simulink model "larix2_tuner_closedLoop"  (R2020b)
settings: Solver=FixedStepDiscrete  StartTime=0.0  StopTime=20  FixedStep=0.002  RelTol=1e-3
PostLoadFcn:
  | load('ThrustTable.mat');
  | init();
values from neighbouring files (symbols this model uses):
  blimp = inertias()    [init.m]
  eul_0 = [-45*pi/180 0 0]    [init.m]
  FLRS3_0 = [0 0 0 0]    [init.m]
  g = 9.810    (= 9.81)    [init.m]
  omega_0 = [0 0 0]    [init.m]
  pos_0 = [0 0 0]    [init.m]
  vel_0 = [0 0 0]    [init.m]
undefined symbols (not defined in the file or in its folder): DiscIntNeverNeededParam
libraries: slpidlib x10, simulink x10, sharedtransform x3, vrlib x3
(part 1 of 2)
settings Model: Creator=ac114611  LastModifiedBy=wendelin
settings DataIOCC: ExternalInput=getinputstruct(op_hover)  InitialState=getstatestruct(op_hover)  ReturnWorkspaceOutputs=off
settings OptimizationCC: DefaultParameterBehavior=Inlined  EnhancedBackFolding=on  PassReuseOutputArgsAs=Individual arguments  MaxStackSize=64  OptimizeBlockOrder=speed  DifferentSizesBufferReuse=on  EfficientTunableParamExpr=on
settings DebuggingCC: ParameterPrecisionLossMsg=none  ParameterTunabilityLossMsg=error  ArithmeticOperatorsInVariantConditions=warning
settings HardwareCC: ProdBitPerPointer=32  ProdBitPerSizeT=32  ProdBitPerPtrDiffT=32  ProdLargestAtomicInteger=Long  ProdLargestAtomicFloat=Double  ProdWordSize=32  ProdHWDeviceType=ARM Compatible->ARM Cortex  TargetBitPerLong=64  TargetBitPerPointer=64  TargetBitPerSizeT=64  TargetBitPerPtrDiffT=64  TargetLongLongMode=on  TargetIntDivRoundTo=Zero  TargetEndianess=LittleEndian  TargetWordSize=64  TargetHWDeviceType=MATLAB Host  ProdEqTarget=off
settings SFSimCC: SimUseLocalCustomCode=off  MATLABDynamicMemAlloc=off  CustomCodeUndefinedFunction=UseInterfaceOnly
settings RTWCC: Description=Embedded Coder  SystemTargetFile=ert.tlc  GenCodeOnly=on  PackageName=larix2_codegen.zip  TemplateMakefile=ert_default_tmf  RTWUseLocalCustomCode=off  Toolchain=GNU gcc/g++ | gmake (64-bit Linux)  IncludeHyperlinkInReport=on  GenerateCodeMetricsReport=on
settings CodeAppCC: ForceParamTrailComments=on  IgnoreCustomStorageClasses=off  OperatorAnnotations=on  SimulinkDataObjDesc=on  SFDataObjDesc=on  InsertBlockDesc=on
settings ERTTargetCC: TargetLangStandard=C99 (ISO)  InlinedParameterPlacement=NonHierarchical  ERTCustomFileTemplate=example_file_process.tlc

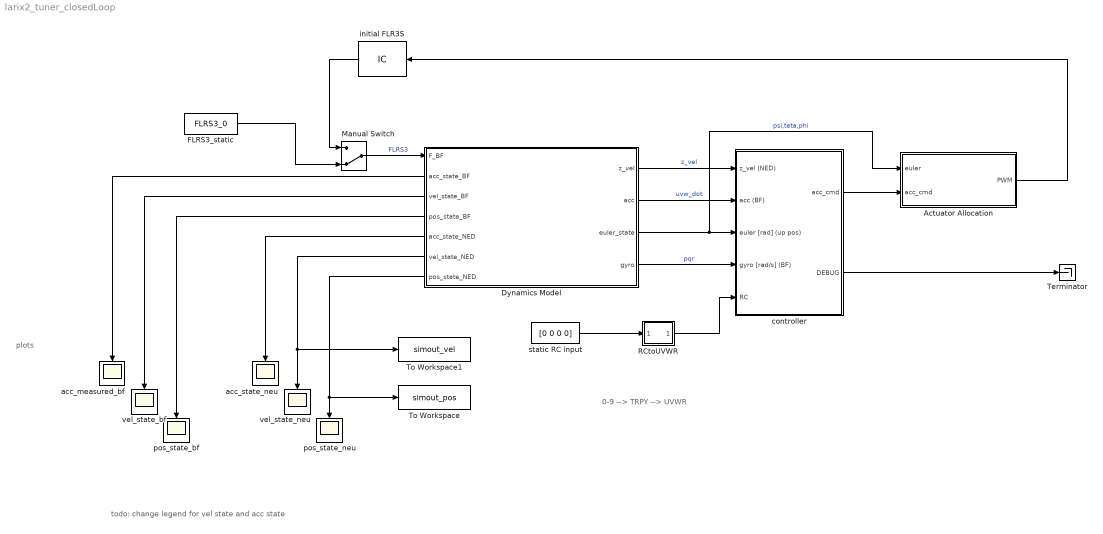
== system larix2_tuner_closedLoop ==
  note: todo: change legend for vel state and acc state
  note: plots
  note: 0-9 --> TRPY --> UVWR
  Actuator Allocation : Subsystem
  Dynamics Model : Subsystem
      settings: PortSchema="{\"entries\":[{\"content\":{\"sides\":[{\"content\":{\"connectorIds\":[\"In1\",\"Out5\",\"Out6\",\"Out7\",\"Out8\",\"Out9\",\"Out10\"]},\"type\":\"ConnectorPlacement.EquallySpacedRectSide\",\"uuid\":\"7b482eda-451f-4705-a72e-674db1e2ea8f\"},{\"content\":{\"connectorIds\":[\"Out1\",\"Out2\",\"Out3\",\"Out4\"],\"side\":\"RIGHT\"},\"type\":\"ConnectorPlacement.EquallySpacedRectSide\",\"uuid\":\"2344d3e9-2a2c-4bd3-8790-1f9d37abcd4c\"},{\"content\":{\"connectorIds\":[],\"side\":\"TOP\"},\"type\":\"ConnectorPlacement.EquallySpacedRectSide\",\"uuid\":\"13a22bb4-0a82-4477-a366-02f381e5ef07\"},{\"content\":{\"connectorIds\":[],\"side\":\"BOTTOM\"},\"type\":\"ConnectorPlacement.EquallySpacedRectSide\",\"uuid\":\"663825dc-fe4c-484f-87e0-eae3c1c76089\"},{\"content\":{\"connectorIds\":[],\"side\":\"HIDDEN\"},\"type\":\"ConnectorPlacement.EquallySpacedRectSide\",\"uuid\":\"0874c0d1-0ac2-489a-adcf-241d9ac40396\"}]},\"type\":\"ConnectorPlacement.EquallySpacedConnector\",\"uuid\":\"4f633129-49ae-43ab-aa97-bf1abe451306\"}],\"packageUris\":[\"http://schema.mathworks.com/mf0/Connector/R2020b\"],\"version\":\"1.0\"}"
  FLRS3_static : Constant  Value=FLRS3_0
  Manual Switch : ManualSwitch  CurrentSetting=0
  RCtoUVWR : Subsystem
  Terminator : Terminator
  To Workspace : ToWorkspace  VariableName=simout_pos  SaveFormat=Structure With Time  SampleTime=-1
  To Workspace1 : ToWorkspace  VariableName=simout_vel  SaveFormat=Structure With Time  SampleTime=-1
  acc_measured_bf : Scope
  acc_state_neu : Scope
  controller : Subsystem
  initial FLR3S : InitialCondition  Value=FLRS3_0
  pos_state_bf : Scope
  pos_state_neu : Scope
  static RC input : Constant  Value=[0 0 0 0]
  vel_state_bf : Scope
  vel_state_neu : Scope
  wires:
  Dynamics Model/4(gyro) -> controller/4(gyro [rad/s] (BF))  "pqr"
  Dynamics Model/2(acc) -> controller/2(acc (BF))  "uvw_dot"
  Dynamics Model/1(z_vel) -> controller/1(z_vel (NED))  "z_vel"
  Dynamics Model/3(euler_state) -> Actuator Allocation/1(euler), controller/3(euler [rad] (up pos))  "psi,teta,phi"
  Dynamics Model/6(vel_state_BF) -> vel_state_bf/1
  Dynamics Model/9(vel_state_NED) -> vel_state_neu/1, To Workspace1/1
  Dynamics Model/10(pos_state_NED) -> pos_state_neu/1, To Workspace/1
  Manual Switch/1 -> Dynamics Model/1(F_BF)  "FLRS3"
  FLRS3_static/1 -> Manual Switch/2
  initial FLR3S/1 -> Manual Switch/1
  Dynamics Model/5(acc_state_BF) -> acc_measured_bf/1
  Dynamics Model/7(pos_state_BF) -> pos_state_bf/1
  static RC input/1 -> RCtoUVWR/1(RC)
  Actuator Allocation/1(PWM) -> initial FLR3S/1
  Dynamics Model/8(acc_state_NED) -> acc_state_neu/1
  controller/2(DEBUG) -> Terminator/1
  controller/1(acc_cmd) -> Actuator Allocation/2(acc_cmd)
  RCtoUVWR/1(Out1) -> controller/5(RC)

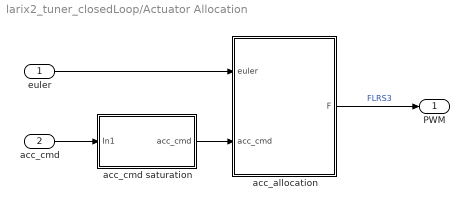
== system larix2_tuner_closedLoop/Actuator Allocation ==
  euler : Inport
  acc_cmd : Inport  Port=2
  acc_allocation : MATLAB Function  TreatAsAtomicUnit=on
  acc_cmd saturation : Subsystem
  PWM : Outport
  wires:
  acc_cmd/1 -> acc_cmd saturation/1(In1)
  acc_cmd saturation/1(acc_cmd) -> acc_allocation/2(acc_cmd)
  euler/1 -> acc_allocation/1(euler)
  acc_allocation/1(F) -> PWM/1  "FLRS3"

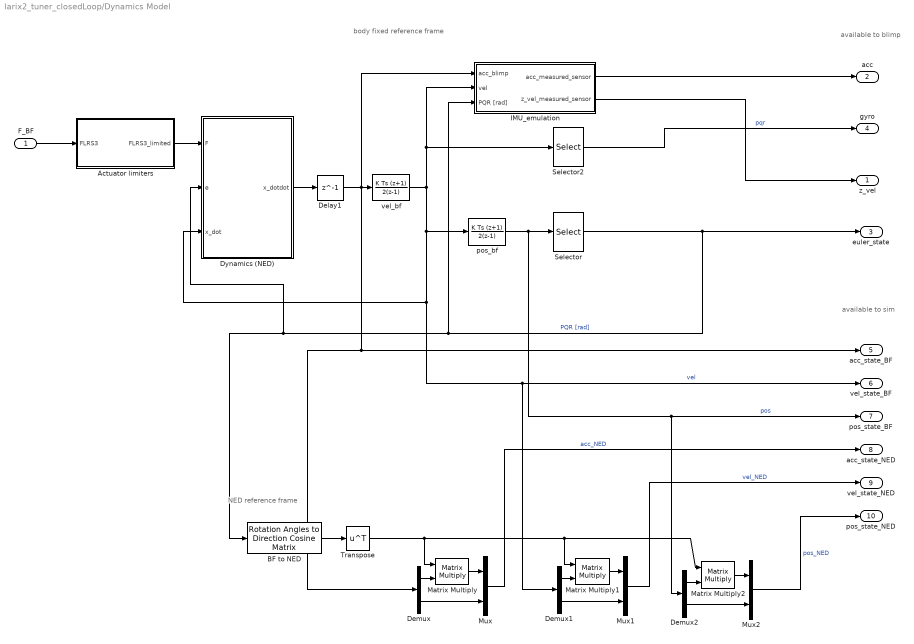
== system larix2_tuner_closedLoop/Dynamics Model ==
  note: NED reference frame
  note: body fixed reference frame
  note: available
      | to sim
  note: available
      | to blimp
  F_BF : Inport
  " BF to NED" : sharedtransform/Rotation Angles to Direction Cosine Matrix  rotationOrder=XYZ  aMode=aMode
      settings: SourceProductBaseCode=AE,PW,MT,UV,VE,VP
  Actuator limiters : Subsystem
  Delay1 : Delay  DelayLength=1  StateName=acceleration_ned
  Demux : Demux  Outputs=2
  Demux1 : Demux  Outputs=2
  Demux2 : Demux  Outputs=2
  Dynamics (NED) : MATLAB Function  TreatAsAtomicUnit=on
  IMU_emulation : Subsystem
  Matrix Multiply : Product  Multiplication=Matrix(*)
  Matrix Multiply1 : Product  Multiplication=Matrix(*)
  Matrix Multiply2 : Product  Multiplication=Matrix(*)
  Mux : Mux  Inputs=2
  Mux1 : Mux  Inputs=2
  Mux2 : Mux  Inputs=2
  Selector : Selector  InputPortWidth=6  IndexOptions=Index vector (dialog)  Indices=[4 5 6]  OutputSizes=1
  Selector2 : Selector  InputPortWidth=6  IndexOptions=Index vector (dialog)  Indices=[4 5 6]  OutputSizes=1
  Transpose : Math  Operator=transpose  SaturateOnIntegerOverflow=on
  pos_bf : DiscreteIntegrator  IntegratorMethod=Integration: Trapezoidal  InitialCondition=[pos_0,eul_0]  SampleTime=-1  StateName=position_bf  ICPrevOutput=DiscIntNeverNeededParam  ICPrevScaledInput=DiscIntNeverNeededParam
  vel_bf : DiscreteIntegrator  IntegratorMethod=Integration: Trapezoidal  InitialCondition=[vel_0,omega_0]  SampleTime=-1  StateName=velocity_bf  ICPrevOutput=DiscIntNeverNeededParam  ICPrevScaledInput=DiscIntNeverNeededParam
  z_vel : Outport  OutDataTypeStr=double
  acc : Outport  Port=2  OutDataTypeStr=double
  euler_state : Outport  Port=3  OutDataTypeStr=double
  gyro : Outport  Port=4  OutDataTypeStr=double
  acc_state_BF : Outport  Port=5
  vel_state_BF : Outport  Port=6  OutDataTypeStr=double
  pos_state_BF : Outport  Port=7
  acc_state_NED : Outport  Port=8
  vel_state_NED : Outport  Port=9
  pos_state_NED : Outport  Port=10
  wires:
  pos_bf/1 -> Demux2/1, pos_state_BF/1, Selector/1  "pos"
  vel_bf/1 -> pos_bf/1, Demux1/1, vel_state_BF/1, Dynamics (NED)/3(x_dot), Selector2/1, IMU_emulation/2(vel)  "vel"
  F_BF/1 -> Actuator limiters/1(FLRS3)
  Dynamics (NED)/1(x_dotdot) -> Delay1/1
  Selector2/1 -> gyro/1  "pqr"
  Mux2/1 -> pos_state_NED/1  "pos_NED"
  Demux/1 -> Matrix Multiply/2
  Demux/2 -> Mux/2
  Matrix Multiply/1 -> Mux/1
  Selector/1 -> Dynamics (NED)/2(e), " BF to NED"/1, IMU_emulation/3(PQR [rad]), euler_state/1  "PQR [rad]"
  Mux/1 -> acc_state_NED/1  "acc_NED"
  Mux1/1 -> vel_state_NED/1  "vel_NED"
  Delay1/1 -> Demux/1, acc_state_BF/1, vel_bf/1, IMU_emulation/1(acc_blimp)
  IMU_emulation/2(z_vel_measured_sensor) -> z_vel/1
  IMU_emulation/1(acc_measured_sensor) -> acc/1
  Demux1/1 -> Matrix Multiply1/2
  Demux1/2 -> Mux1/2
  Matrix Multiply1/1 -> Mux1/1
  Demux2/2 -> Mux2/2
  Demux2/1 -> Matrix Multiply2/2
  Matrix Multiply2/1 -> Mux2/1
  Actuator limiters/1(FLRS3_limited) -> Dynamics (NED)/1(F)
  " BF to NED"/1 -> Transpose/1
  Transpose/1 -> Matrix Multiply/1, Matrix Multiply1/1, Matrix Multiply2/1

== system larix2_tuner_closedLoop/RCtoUVWR ==
  note: uv_dot_max
      | wr_max
  note: 0-9 --> TRPY --> UVWR
  RC : Inport
  RC input safety : Subsystem
  uvwr_max : Gain  Gain=single([blimp.prp.du_input_max, blimp.prp.dv_input_max, blimp.prp.w_input_max, blimp.prp.r_input_max])
  Out1 : Outport
  wires:
  RC input safety/1(Out1) -> uvwr_max/1
  RC/1 -> RC input safety/1(RC)
  uvwr_max/1 -> Out1/1  "uvwr.desired [m/s]"

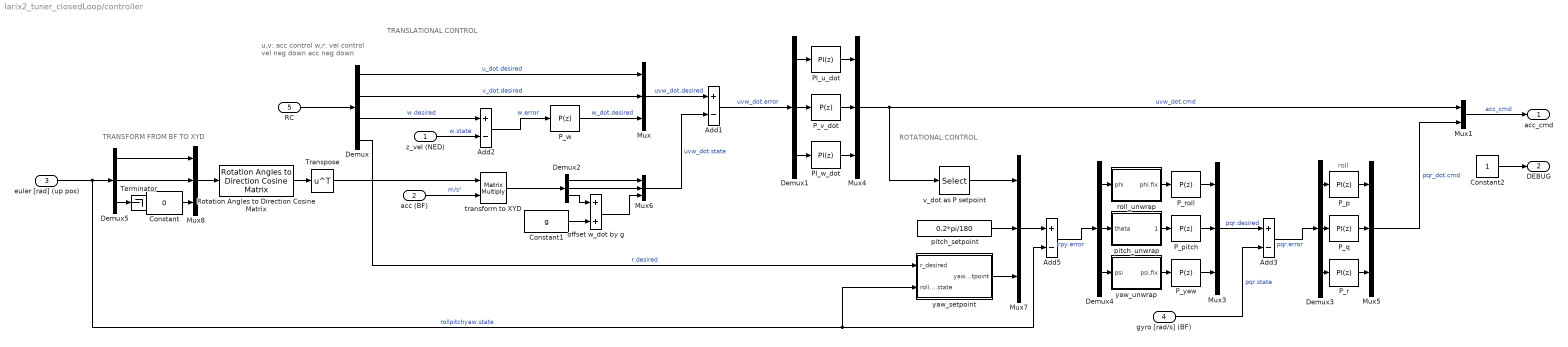
== system larix2_tuner_closedLoop/controller ==
  note: roll
  note: TRANSFORM FROM BF TO XYD
  note: u,v: acc control
      | w,r: vel control
      |
      | vel neg down
      | acc neg down
  note: TRANSLATIONAL CONTROL
  note: ROTATIONAL CONTROL
  z_vel (NED) : Inport  PortDimensions=1
  acc (BF) : Inport  Port=2  PortDimensions=3
  euler [rad] (up pos) : Inport  Port=3  PortDimensions=3
  gyro [rad/s] (BF) : Inport  Port=4  PortDimensions=3
  RC : Inport  Port=5
  Add{1..3,5} (4 alike) : Sum  Inputs=+-
  Constant : Constant  Value=0
  Constant1 : Constant  Value=g
  Constant2 : Constant
  Demux : Demux
  Demux{1..5} (5 alike) : Demux  Outputs=3
  Mux{,3..8} (7 alike) : Mux  Inputs=3
  Mux1 : Mux  Inputs=2
  PI_u_dot : slpidlib/PID Controller  Controller=PI  Form=Parallel  TimeDomain=Discrete-time  UseExternalTs=off  SampleTime=-1  IntegratorMethod=Trapezoidal  FilterMethod=Forward Euler  ControllerParametersSource=internal  P=1  I=0  D=0  UseFilter=on  N=100  TunerSelectOption=Transfer Function Based (PID Tuner App)  InitialConditionSource=internal  InitialConditionForIntegrator=0  InitialConditionForFilter=0  DifferentiatorICPrevScaledInput=0  ExternalReset=none  TrackingMode=off  Kt=1  LimitOutput=off  SatLimitsSource=internal  UpperSaturationLimit=0.4*g  LowerSaturationLimit=-0.4*g  LinearizeAsGain=off  AntiWindupMode=none  Kb=1  POutMin=[]  POutMax=[]  IOutMin=[]  IOutMax=[]  DOutMin=[]  DOutMax=[]  NOutMin=[]  NOutMax=[]  SumOutMin=[]  SumOutMax=[]  SaturationOutMin=[]  SaturationOutMax=[]  PParamMin=[]  PParamMax=[]  IParamMin=[]  IParamMax=[]  DParamMin=[]  DParamMax=[]  NParamMin=[]  NParamMax=[]  KbParamMin=[]  KbParamMax=[]  KtParamMin=[]  KtParamMax=[]  KbOutMin=[]  KbOutMax=[]  KtOutMin=[]  KtOutMax=[]  IntegratorOutMin=[]  IntegratorOutMax=[]  FilterOutMin=[]  FilterOutMax=[]  SumI1OutMin=[]  SumI1OutMax=[]  SumI2OutMin=[]  SumI2OutMax=[]  SumI3OutMin=[]  SumI3OutMax=[]  SumI4OutMin=[]  SumI4OutMax=[]  SumDOutMin=[]  SumDOutMax=[]  DifferentiatorOutMin=[]  DifferentiatorOutMax=[]  FilterDiffOutCoefMin=[]  FilterDiffOutCoefMax=[]  ReciprocalOutMin=[]  ReciprocalOutMax=[]  SumDenOutMin=[]  SumDenOutMax=[]  SumNumOutMin=[]  SumNumOutMax=[]  DivideOutMin=[]  DivideOutMax=[]  UdiffTsProdOutMin=[]  UdiffTsProdOutMax=[]  NTsProdOutMin=[]  NTsProdOutMax=[]  UintegralTsProdOutMin=[]  UintegralTsProdOutMax=[]  UngainTsProdOutMin=[]  UngainTsProdOutMax=[]  IntegratorContinuousStateAttributes=''  IntegratorStateMustResolveToSignalObject=off  IntegratorRTWStateStorageClass=Auto  FilterContinuousStateAttributes=''  FilterStateMustResolveToSignalObject=off  FilterRTWStateStorageClass=Auto  ParallelPVariant=InternalParameters  IdealPVariant=Disabled  IVariant=InternalParameters  DVariant=Disabled  IntegratorVariant=Discrete  SatVariant=Disabled  AWVariant=Passthrough  PCopyVariant=Disabled  TRVariant=Disabled  FdbkBlocksVariant=Forward  IdealPFdbkVariant=Disabled  SatFdbkVariant=Disabled  DerivativeFilterVariant=Disabled  NVariant=Disabled  NCopyVariant=Disabled_SignalSpec  FilterICVariant=Disabled  IntegratorICVariant=InternalICs  ExternalResetVariant=Disabled  TRSumVariant=Passthrough  SumFdbkVariant=Disabled  SumVariant=Sum_PI  TsampFilterVariant=InternalTs  TsampNgainVariant=Passthrough  TsampIntegralVariant=Passthrough  ExternalSaturationOutDataTypeStr=Inherit: Same as second input
  PI_w_dot : slpidlib/PID Controller  Controller=PI  Form=Parallel  TimeDomain=Discrete-time  UseExternalTs=off  SampleTime=-1  IntegratorMethod=Forward Euler  FilterMethod=Forward Euler  ControllerParametersSource=internal  P=1.8  I=1.4  D=0  UseFilter=on  N=100  TunerSelectOption=Transfer Function Based (PID Tuner App)  InitialConditionSource=internal  InitialConditionForIntegrator=1.1  InitialConditionForFilter=0  DifferentiatorICPrevScaledInput=0  ExternalReset=none  TrackingMode=off  Kt=1  LimitOutput=off  SatLimitsSource=internal  UpperSaturationLimit=inf  LowerSaturationLimit=0  LinearizeAsGain=off  AntiWindupMode=none  Kb=1  POutMin=[]  POutMax=[]  IOutMin=[]  IOutMax=[]  DOutMin=[]  DOutMax=[]  NOutMin=[]  NOutMax=[]  SumOutMin=[]  SumOutMax=[]  SaturationOutMin=[]  SaturationOutMax=[]  PParamMin=[]  PParamMax=[]  IParamMin=[]  IParamMax=[]  DParamMin=[]  DParamMax=[]  NParamMin=[]  NParamMax=[]  KbParamMin=[]  KbParamMax=[]  KtParamMin=[]  KtParamMax=[]  KbOutMin=[]  KbOutMax=[]  KtOutMin=[]  KtOutMax=[]  IntegratorOutMin=[]  IntegratorOutMax=[]  FilterOutMin=[]  FilterOutMax=[]  SumI1OutMin=[]  SumI1OutMax=[]  SumI2OutMin=[]  SumI2OutMax=[]  SumI3OutMin=[]  SumI3OutMax=[]  SumI4OutMin=[]  SumI4OutMax=[]  SumDOutMin=[]  SumDOutMax=[]  DifferentiatorOutMin=[]  DifferentiatorOutMax=[]  FilterDiffOutCoefMin=[]  FilterDiffOutCoefMax=[]  ReciprocalOutMin=[]  ReciprocalOutMax=[]  SumDenOutMin=[]  SumDenOutMax=[]  SumNumOutMin=[]  SumNumOutMax=[]  DivideOutMin=[]  DivideOutMax=[]  UdiffTsProdOutMin=[]  UdiffTsProdOutMax=[]  NTsProdOutMin=[]  NTsProdOutMax=[]  UintegralTsProdOutMin=[]  UintegralTsProdOutMax=[]  UngainTsProdOutMin=[]  UngainTsProdOutMax=[]  IntegratorContinuousStateAttributes=''  IntegratorStateMustResolveToSignalObject=off  IntegratorRTWStateStorageClass=Auto  FilterContinuousStateAttributes=''  FilterStateMustResolveToSignalObject=off  FilterRTWStateStorageClass=Auto  ParallelPVariant=InternalParameters  IdealPVariant=Disabled  IVariant=InternalParameters  DVariant=Disabled  IntegratorVariant=Discrete  SatVariant=Disabled  AWVariant=Passthrough  PCopyVariant=Disabled  TRVariant=Disabled  FdbkBlocksVariant=Forward  IdealPFdbkVariant=Disabled  SatFdbkVariant=Disabled  DerivativeFilterVariant=Disabled  NVariant=Disabled  NCopyVariant=Disabled_SignalSpec  FilterICVariant=Disabled  IntegratorICVariant=InternalICs  ExternalResetVariant=Disabled  TRSumVariant=Passthrough  SumFdbkVariant=Disabled  SumVariant=Sum_PI  TsampFilterVariant=InternalTs  TsampNgainVariant=Passthrough  TsampIntegralVariant=Passthrough  ExternalSaturationOutDataTypeStr=Inherit: Same as second input
  P_p : slpidlib/PID Controller  Controller=PI  Form=Parallel  TimeDomain=Discrete-time  UseExternalTs=off  SampleTime=-1  IntegratorMethod=Forward Euler  FilterMethod=Forward Euler  ControllerParametersSource=internal  P=1  I=0  D=0  UseFilter=on  N=100  TunerSelectOption=Transfer Function Based (PID Tuner App)  InitialConditionSource=internal  InitialConditionForIntegrator=0  InitialConditionForFilter=0  DifferentiatorICPrevScaledInput=0  ExternalReset=none  TrackingMode=off  Kt=1  LimitOutput=off  SatLimitsSource=internal  UpperSaturationLimit=inf  LowerSaturationLimit=-inf  LinearizeAsGain=on  AntiWindupMode=none  Kb=1  POutMin=[]  POutMax=[]  IOutMin=[]  IOutMax=[]  DOutMin=[]  DOutMax=[]  NOutMin=[]  NOutMax=[]  SumOutMin=[]  SumOutMax=[]  SaturationOutMin=[]  SaturationOutMax=[]  PParamMin=[]  PParamMax=[]  IParamMin=[]  IParamMax=[]  DParamMin=[]  DParamMax=[]  NParamMin=[]  NParamMax=[]  KbParamMin=[]  KbParamMax=[]  KtParamMin=[]  KtParamMax=[]  KbOutMin=[]  KbOutMax=[]  KtOutMin=[]  KtOutMax=[]  IntegratorOutMin=[]  IntegratorOutMax=[]  FilterOutMin=[]  FilterOutMax=[]  SumI1OutMin=[]  SumI1OutMax=[]  SumI2OutMin=[]  SumI2OutMax=[]  SumI3OutMin=[]  SumI3OutMax=[]  SumI4OutMin=[]  SumI4OutMax=[]  SumDOutMin=[]  SumDOutMax=[]  DifferentiatorOutMin=[]  DifferentiatorOutMax=[]  FilterDiffOutCoefMin=[]  FilterDiffOutCoefMax=[]  ReciprocalOutMin=[]  ReciprocalOutMax=[]  SumDenOutMin=[]  SumDenOutMax=[]  SumNumOutMin=[]  SumNumOutMax=[]  DivideOutMin=[]  DivideOutMax=[]  UdiffTsProdOutMin=[]  UdiffTsProdOutMax=[]  NTsProdOutMin=[]  NTsProdOutMax=[]  UintegralTsProdOutMin=[]  UintegralTsProdOutMax=[]  UngainTsProdOutMin=[]  UngainTsProdOutMax=[]  IntegratorContinuousStateAttributes=''  IntegratorStateMustResolveToSignalObject=off  IntegratorRTWStateStorageClass=Auto  FilterContinuousStateAttributes=''  FilterStateMustResolveToSignalObject=off  FilterRTWStateStorageClass=Auto  ParallelPVariant=InternalParameters  IdealPVariant=Disabled  IVariant=InternalParameters  DVariant=Disabled  IntegratorVariant=Discrete  SatVariant=Disabled  AWVariant=Passthrough  PCopyVariant=Disabled  TRVariant=Disabled  FdbkBlocksVariant=Forward  IdealPFdbkVariant=Disabled  SatFdbkVariant=Disabled  DerivativeFilterVariant=Disabled  NVariant=Disabled  NCopyVariant=Disabled_SignalSpec  FilterICVariant=Disabled  IntegratorICVariant=InternalICs  ExternalResetVariant=Disabled  TRSumVariant=Passthrough  SumFdbkVariant=Disabled  SumVariant=Sum_PI  TsampFilterVariant=InternalTs  TsampNgainVariant=Passthrough  TsampIntegralVariant=Passthrough  ExternalSaturationOutDataTypeStr=Inherit: Same as second input
  P_pitch : slpidlib/PID Controller  Controller=P  Form=Parallel  TimeDomain=Discrete-time  UseExternalTs=off  SampleTime=-1  IntegratorMethod=Forward Euler  FilterMethod=Forward Euler  ControllerParametersSource=internal  P=1  I=0  D=0  UseFilter=on  N=100  TunerSelectOption=Transfer Function Based (PID Tuner App)  InitialConditionSource=internal  InitialConditionForIntegrator=0  InitialConditionForFilter=0  DifferentiatorICPrevScaledInput=0  ExternalReset=none  TrackingMode=off  Kt=1  LimitOutput=off  SatLimitsSource=internal  UpperSaturationLimit=inf  LowerSaturationLimit=-inf  LinearizeAsGain=on  AntiWindupMode=none  Kb=1  POutMin=[]  POutMax=[]  IOutMin=[]  IOutMax=[]  DOutMin=[]  DOutMax=[]  NOutMin=[]  NOutMax=[]  SumOutMin=[]  SumOutMax=[]  SaturationOutMin=[]  SaturationOutMax=[]  PParamMin=[]  PParamMax=[]  IParamMin=[]  IParamMax=[]  DParamMin=[]  DParamMax=[]  NParamMin=[]  NParamMax=[]  KbParamMin=[]  KbParamMax=[]  KtParamMin=[]  KtParamMax=[]  KbOutMin=[]  KbOutMax=[]  KtOutMin=[]  KtOutMax=[]  IntegratorOutMin=[]  IntegratorOutMax=[]  FilterOutMin=[]  FilterOutMax=[]  SumI1OutMin=[]  SumI1OutMax=[]  SumI2OutMin=[]  SumI2OutMax=[]  SumI3OutMin=[]  SumI3OutMax=[]  SumI4OutMin=[]  SumI4OutMax=[]  SumDOutMin=[]  SumDOutMax=[]  DifferentiatorOutMin=[]  DifferentiatorOutMax=[]  FilterDiffOutCoefMin=[]  FilterDiffOutCoefMax=[]  ReciprocalOutMin=[]  ReciprocalOutMax=[]  SumDenOutMin=[]  SumDenOutMax=[]  SumNumOutMin=[]  SumNumOutMax=[]  DivideOutMin=[]  DivideOutMax=[]  UdiffTsProdOutMin=[]  UdiffTsProdOutMax=[]  NTsProdOutMin=[]  NTsProdOutMax=[]  UintegralTsProdOutMin=[]  UintegralTsProdOutMax=[]  UngainTsProdOutMin=[]  UngainTsProdOutMax=[]  IntegratorContinuousStateAttributes=''  IntegratorStateMustResolveToSignalObject=off  IntegratorRTWStateStorageClass=Auto  FilterContinuousStateAttributes=''  FilterStateMustResolveToSignalObject=off  FilterRTWStateStorageClass=Auto  ParallelPVariant=InternalParameters  IdealPVariant=Disabled  IVariant=Disabled  DVariant=Disabled  IntegratorVariant=Disabled  SatVariant=Disabled  AWVariant=Disabled  PCopyVariant=Disabled  TRVariant=Disabled  FdbkBlocksVariant=Forward  IdealPFdbkVariant=Disabled  SatFdbkVariant=Disabled  DerivativeFilterVariant=Disabled  NVariant=Disabled  NCopyVariant=Disabled_SignalSpec  FilterICVariant=Disabled  IntegratorICVariant=Disabled  ExternalResetVariant=Disabled  TRSumVariant=Passthrough  SumFdbkVariant=Disabled  SumVariant=Passthrough_P  TsampFilterVariant=InternalTs  TsampNgainVariant=Passthrough  TsampIntegralVariant=Disabled_SignalSpec  ExternalSaturationOutDataTypeStr=Inherit: Same as second input
  P_q : slpidlib/PID Controller  Controller=PI  Form=Parallel  TimeDomain=Discrete-time  UseExternalTs=off  SampleTime=-1  IntegratorMethod=Forward Euler  FilterMethod=Forward Euler  ControllerParametersSource=internal  P=1  I=0  D=0  UseFilter=on  N=100  TunerSelectOption=Transfer Function Based (PID Tuner App)  InitialConditionSource=internal  InitialConditionForIntegrator=0  InitialConditionForFilter=0  DifferentiatorICPrevScaledInput=0  ExternalReset=none  TrackingMode=off  Kt=1  LimitOutput=off  SatLimitsSource=internal  UpperSaturationLimit=inf  LowerSaturationLimit=-inf  LinearizeAsGain=on  AntiWindupMode=none  Kb=1  POutMin=[]  POutMax=[]  IOutMin=[]  IOutMax=[]  DOutMin=[]  DOutMax=[]  NOutMin=[]  NOutMax=[]  SumOutMin=[]  SumOutMax=[]  SaturationOutMin=[]  SaturationOutMax=[]  PParamMin=[]  PParamMax=[]  IParamMin=[]  IParamMax=[]  DParamMin=[]  DParamMax=[]  NParamMin=[]  NParamMax=[]  KbParamMin=[]  KbParamMax=[]  KtParamMin=[]  KtParamMax=[]  KbOutMin=[]  KbOutMax=[]  KtOutMin=[]  KtOutMax=[]  IntegratorOutMin=[]  IntegratorOutMax=[]  FilterOutMin=[]  FilterOutMax=[]  SumI1OutMin=[]  SumI1OutMax=[]  SumI2OutMin=[]  SumI2OutMax=[]  SumI3OutMin=[]  SumI3OutMax=[]  SumI4OutMin=[]  SumI4OutMax=[]  SumDOutMin=[]  SumDOutMax=[]  DifferentiatorOutMin=[]  DifferentiatorOutMax=[]  FilterDiffOutCoefMin=[]  FilterDiffOutCoefMax=[]  ReciprocalOutMin=[]  ReciprocalOutMax=[]  SumDenOutMin=[]  SumDenOutMax=[]  SumNumOutMin=[]  SumNumOutMax=[]  DivideOutMin=[]  DivideOutMax=[]  UdiffTsProdOutMin=[]  UdiffTsProdOutMax=[]  NTsProdOutMin=[]  NTsProdOutMax=[]  UintegralTsProdOutMin=[]  UintegralTsProdOutMax=[]  UngainTsProdOutMin=[]  UngainTsProdOutMax=[]  IntegratorContinuousStateAttributes=''  IntegratorStateMustResolveToSignalObject=off  IntegratorRTWStateStorageClass=Auto  FilterContinuousStateAttributes=''  FilterStateMustResolveToSignalObject=off  FilterRTWStateStorageClass=Auto  ParallelPVariant=InternalParameters  IdealPVariant=Disabled  IVariant=InternalParameters  DVariant=Disabled  IntegratorVariant=Discrete  SatVariant=Disabled  AWVariant=Passthrough  PCopyVariant=Disabled  TRVariant=Disabled  FdbkBlocksVariant=Forward  IdealPFdbkVariant=Disabled  SatFdbkVariant=Disabled  DerivativeFilterVariant=Disabled  NVariant=Disabled  NCopyVariant=Disabled_SignalSpec  FilterICVariant=Disabled  IntegratorICVariant=InternalICs  ExternalResetVariant=Disabled  TRSumVariant=Passthrough  SumFdbkVariant=Disabled  SumVariant=Sum_PI  TsampFilterVariant=InternalTs  TsampNgainVariant=Passthrough  TsampIntegralVariant=Passthrough  ExternalSaturationOutDataTypeStr=Inherit: Same as second input
  P_r : slpidlib/PID Controller  Controller=PI  Form=Parallel  TimeDomain=Discrete-time  UseExternalTs=off  SampleTime=-1  IntegratorMethod=Forward Euler  FilterMethod=Forward Euler  ControllerParametersSource=internal  P=0.7  I=0.5  D=0  UseFilter=on  N=100  TunerSelectOption=Transfer Function Based (PID Tuner App)  InitialConditionSource=internal  InitialConditionForIntegrator=0  InitialConditionForFilter=0  DifferentiatorICPrevScaledInput=0  ExternalReset=none  TrackingMode=off  Kt=1  LimitOutput=off  SatLimitsSource=internal  UpperSaturationLimit=inf  LowerSaturationLimit=-inf  LinearizeAsGain=on  AntiWindupMode=none  Kb=1  POutMin=[]  POutMax=[]  IOutMin=[]  IOutMax=[]  DOutMin=[]  DOutMax=[]  NOutMin=[]  NOutMax=[]  SumOutMin=[]  SumOutMax=[]  SaturationOutMin=[]  SaturationOutMax=[]  PParamMin=[]  PParamMax=[]  IParamMin=[]  IParamMax=[]  DParamMin=[]  DParamMax=[]  NParamMin=[]  NParamMax=[]  KbParamMin=[]  KbParamMax=[]  KtParamMin=[]  KtParamMax=[]  KbOutMin=[]  KbOutMax=[]  KtOutMin=[]  KtOutMax=[]  IntegratorOutMin=[]  IntegratorOutMax=[]  FilterOutMin=[]  FilterOutMax=[]  SumI1OutMin=[]  SumI1OutMax=[]  SumI2OutMin=[]  SumI2OutMax=[]  SumI3OutMin=[]  SumI3OutMax=[]  SumI4OutMin=[]  SumI4OutMax=[]  SumDOutMin=[]  SumDOutMax=[]  DifferentiatorOutMin=[]  DifferentiatorOutMax=[]  FilterDiffOutCoefMin=[]  FilterDiffOutCoefMax=[]  ReciprocalOutMin=[]  ReciprocalOutMax=[]  SumDenOutMin=[]  SumDenOutMax=[]  SumNumOutMin=[]  SumNumOutMax=[]  DivideOutMin=[]  DivideOutMax=[]  UdiffTsProdOutMin=[]  UdiffTsProdOutMax=[]  NTsProdOutMin=[]  NTsProdOutMax=[]  UintegralTsProdOutMin=[]  UintegralTsProdOutMax=[]  UngainTsProdOutMin=[]  UngainTsProdOutMax=[]  IntegratorContinuousStateAttributes=''  IntegratorStateMustResolveToSignalObject=off  IntegratorRTWStateStorageClass=Auto  FilterContinuousStateAttributes=''  FilterStateMustResolveToSignalObject=off  FilterRTWStateStorageClass=Auto  ParallelPVariant=InternalParameters  IdealPVariant=Disabled  IVariant=InternalParameters  DVariant=Disabled  IntegratorVariant=Discrete  SatVariant=Disabled  AWVariant=Passthrough  PCopyVariant=Disabled  TRVariant=Disabled  FdbkBlocksVariant=Forward  IdealPFdbkVariant=Disabled  SatFdbkVariant=Disabled  DerivativeFilterVariant=Disabled  NVariant=Disabled  NCopyVariant=Disabled_SignalSpec  FilterICVariant=Disabled  IntegratorICVariant=InternalICs  ExternalResetVariant=Disabled  TRSumVariant=Passthrough  SumFdbkVariant=Disabled  SumVariant=Sum_PI  TsampFilterVariant=InternalTs  TsampNgainVariant=Passthrough  TsampIntegralVariant=Passthrough  ExternalSaturationOutDataTypeStr=Inherit: Same as second input
  P_roll : slpidlib/PID Controller  Controller=P  Form=Parallel  TimeDomain=Discrete-time  UseExternalTs=off  SampleTime=-1  IntegratorMethod=Forward Euler  FilterMethod=Forward Euler  ControllerParametersSource=internal  P=0  I=0  D=0  UseFilter=on  N=100  TunerSelectOption=Transfer Function Based (PID Tuner App)  InitialConditionSource=internal  InitialConditionForIntegrator=0  InitialConditionForFilter=0  DifferentiatorICPrevScaledInput=0  ExternalReset=none  TrackingMode=off  Kt=1  LimitOutput=off  SatLimitsSource=internal  UpperSaturationLimit=inf  LowerSaturationLimit=-inf  LinearizeAsGain=on  AntiWindupMode=none  Kb=1  POutMin=[]  POutMax=[]  IOutMin=[]  IOutMax=[]  DOutMin=[]  DOutMax=[]  NOutMin=[]  NOutMax=[]  SumOutMin=[]  SumOutMax=[]  SaturationOutMin=[]  SaturationOutMax=[]  PParamMin=[]  PParamMax=[]  IParamMin=[]  IParamMax=[]  DParamMin=[]  DParamMax=[]  NParamMin=[]  NParamMax=[]  KbParamMin=[]  KbParamMax=[]  KtParamMin=[]  KtParamMax=[]  KbOutMin=[]  KbOutMax=[]  KtOutMin=[]  KtOutMax=[]  IntegratorOutMin=[]  IntegratorOutMax=[]  FilterOutMin=[]  FilterOutMax=[]  SumI1OutMin=[]  SumI1OutMax=[]  SumI2OutMin=[]  SumI2OutMax=[]  SumI3OutMin=[]  SumI3OutMax=[]  SumI4OutMin=[]  SumI4OutMax=[]  SumDOutMin=[]  SumDOutMax=[]  DifferentiatorOutMin=[]  DifferentiatorOutMax=[]  FilterDiffOutCoefMin=[]  FilterDiffOutCoefMax=[]  ReciprocalOutMin=[]  ReciprocalOutMax=[]  SumDenOutMin=[]  SumDenOutMax=[]  SumNumOutMin=[]  SumNumOutMax=[]  DivideOutMin=[]  DivideOutMax=[]  UdiffTsProdOutMin=[]  UdiffTsProdOutMax=[]  NTsProdOutMin=[]  NTsProdOutMax=[]  UintegralTsProdOutMin=[]  UintegralTsProdOutMax=[]  UngainTsProdOutMin=[]  UngainTsProdOutMax=[]  IntegratorContinuousStateAttributes=''  IntegratorStateMustResolveToSignalObject=off  IntegratorRTWStateStorageClass=Auto  FilterContinuousStateAttributes=''  FilterStateMustResolveToSignalObject=off  FilterRTWStateStorageClass=Auto  ParallelPVariant=InternalParameters  IdealPVariant=Disabled  IVariant=Disabled  DVariant=Disabled  IntegratorVariant=Disabled  SatVariant=Disabled  AWVariant=Disabled  PCopyVariant=Disabled  TRVariant=Disabled  FdbkBlocksVariant=Forward  IdealPFdbkVariant=Disabled  SatFdbkVariant=Disabled  DerivativeFilterVariant=Disabled  NVariant=Disabled  NCopyVariant=Disabled_SignalSpec  FilterICVariant=Disabled  IntegratorICVariant=Disabled  ExternalResetVariant=Disabled  TRSumVariant=Passthrough  SumFdbkVariant=Disabled  SumVariant=Passthrough_P  TsampFilterVariant=InternalTs  TsampNgainVariant=Passthrough  TsampIntegralVariant=Disabled_SignalSpec  ExternalSaturationOutDataTypeStr=Inherit: Same as second input
  P_v_dot : slpidlib/PID Controller  Controller=P  Form=Parallel  TimeDomain=Discrete-time  UseExternalTs=off  SampleTime=-1  IntegratorMethod=Forward Euler  FilterMethod=Forward Euler  ControllerParametersSource=internal  P=2.5 *pi/180  I=1  D=0  UseFilter=on  N=100  TunerSelectOption=Transfer Function Based (PID Tuner App)  InitialConditionSource=internal  InitialConditionForIntegrator=0  InitialConditionForFilter=0  DifferentiatorICPrevScaledInput=0  ExternalReset=none  TrackingMode=off  Kt=1  LimitOutput=off  SatLimitsSource=internal  UpperSaturationLimit=inf  LowerSaturationLimit=-inf  LinearizeAsGain=on  AntiWindupMode=none  Kb=1  POutMin=[]  POutMax=[]  IOutMin=[]  IOutMax=[]  DOutMin=[]  DOutMax=[]  NOutMin=[]  NOutMax=[]  SumOutMin=[]  SumOutMax=[]  SaturationOutMin=[]  SaturationOutMax=[]  PParamMin=[]  PParamMax=[]  IParamMin=[]  IParamMax=[]  DParamMin=[]  DParamMax=[]  NParamMin=[]  NParamMax=[]  KbParamMin=[]  KbParamMax=[]  KtParamMin=[]  KtParamMax=[]  KbOutMin=[]  KbOutMax=[]  KtOutMin=[]  KtOutMax=[]  IntegratorOutMin=[]  IntegratorOutMax=[]  FilterOutMin=[]  FilterOutMax=[]  SumI1OutMin=[]  SumI1OutMax=[]  SumI2OutMin=[]  SumI2OutMax=[]  SumI3OutMin=[]  SumI3OutMax=[]  SumI4OutMin=[]  SumI4OutMax=[]  SumDOutMin=[]  SumDOutMax=[]  DifferentiatorOutMin=[]  DifferentiatorOutMax=[]  FilterDiffOutCoefMin=[]  FilterDiffOutCoefMax=[]  ReciprocalOutMin=[]  ReciprocalOutMax=[]  SumDenOutMin=[]  SumDenOutMax=[]  SumNumOutMin=[]  SumNumOutMax=[]  DivideOutMin=[]  DivideOutMax=[]  UdiffTsProdOutMin=[]  UdiffTsProdOutMax=[]  NTsProdOutMin=[]  NTsProdOutMax=[]  UintegralTsProdOutMin=[]  UintegralTsProdOutMax=[]  UngainTsProdOutMin=[]  UngainTsProdOutMax=[]  IntegratorContinuousStateAttributes=''  IntegratorStateMustResolveToSignalObject=off  IntegratorRTWStateStorageClass=Auto  FilterContinuousStateAttributes=''  FilterStateMustResolveToSignalObject=off  FilterRTWStateStorageClass=Auto  ParallelPVariant=InternalParameters  IdealPVariant=Disabled  IVariant=Disabled  DVariant=Disabled  IntegratorVariant=Disabled  SatVariant=Disabled  AWVariant=Disabled  PCopyVariant=Disabled  TRVariant=Disabled  FdbkBlocksVariant=Forward  IdealPFdbkVariant=Disabled  SatFdbkVariant=Disabled  DerivativeFilterVariant=Disabled  NVariant=Disabled  NCopyVariant=Disabled_SignalSpec  FilterICVariant=Disabled  IntegratorICVariant=Disabled  ExternalResetVariant=Disabled  TRSumVariant=Passthrough  SumFdbkVariant=Disabled  SumVariant=Passthrough_P  TsampFilterVariant=InternalTs  TsampNgainVariant=Passthrough  TsampIntegralVariant=Disabled_SignalSpec  ExternalSaturationOutDataTypeStr=Inherit: Same as second input
  P_w : slpidlib/PID Controller  Controller=P  Form=Parallel  TimeDomain=Discrete-time  UseExternalTs=off  SampleTime=-1  IntegratorMethod=Forward Euler  FilterMethod=Forward Euler  ControllerParametersSource=internal  P=1.3  I=0  D=0  UseFilter=on  N=100  TunerSelectOption=Transfer Function Based (PID Tuner App)  InitialConditionSource=internal  InitialConditionForIntegrator=0  InitialConditionForFilter=0  DifferentiatorICPrevScaledInput=0  ExternalReset=none  TrackingMode=off  Kt=1  LimitOutput=off  SatLimitsSource=internal  UpperSaturationLimit=inf  LowerSaturationLimit=-inf  LinearizeAsGain=off  AntiWindupMode=none  Kb=1  POutMin=[]  POutMax=[]  IOutMin=[]  IOutMax=[]  DOutMin=[]  DOutMax=[]  NOutMin=[]  NOutMax=[]  SumOutMin=[]  SumOutMax=[]  SaturationOutMin=[]  SaturationOutMax=[]  PParamMin=[]  PParamMax=[]  IParamMin=[]  IParamMax=[]  DParamMin=[]  DParamMax=[]  NParamMin=[]  NParamMax=[]  KbParamMin=[]  KbParamMax=[]  KtParamMin=[]  KtParamMax=[]  KbOutMin=[]  KbOutMax=[]  KtOutMin=[]  KtOutMax=[]  IntegratorOutMin=[]  IntegratorOutMax=[]  FilterOutMin=[]  FilterOutMax=[]  SumI1OutMin=[]  SumI1OutMax=[]  SumI2OutMin=[]  SumI2OutMax=[]  SumI3OutMin=[]  SumI3OutMax=[]  SumI4OutMin=[]  SumI4OutMax=[]  SumDOutMin=[]  SumDOutMax=[]  DifferentiatorOutMin=[]  DifferentiatorOutMax=[]  FilterDiffOutCoefMin=[]  FilterDiffOutCoefMax=[]  ReciprocalOutMin=[]  ReciprocalOutMax=[]  SumDenOutMin=[]  SumDenOutMax=[]  SumNumOutMin=[]  SumNumOutMax=[]  DivideOutMin=[]  DivideOutMax=[]  UdiffTsProdOutMin=[]  UdiffTsProdOutMax=[]  NTsProdOutMin=[]  NTsProdOutMax=[]  UintegralTsProdOutMin=[]  UintegralTsProdOutMax=[]  UngainTsProdOutMin=[]  UngainTsProdOutMax=[]  IntegratorContinuousStateAttributes=''  IntegratorStateMustResolveToSignalObject=off  IntegratorRTWStateStorageClass=Auto  FilterContinuousStateAttributes=''  FilterStateMustResolveToSignalObject=off  FilterRTWStateStorageClass=Auto  ParallelPVariant=InternalParameters  IdealPVariant=Disabled  IVariant=Disabled  DVariant=Disabled  IntegratorVariant=Disabled  SatVariant=Disabled  AWVariant=Disabled  PCopyVariant=Disabled  TRVariant=Disabled  FdbkBlocksVariant=Forward  IdealPFdbkVariant=Disabled  SatFdbkVariant=Disabled  DerivativeFilterVariant=Disabled  NVariant=Disabled  NCopyVariant=Disabled_SignalSpec  FilterICVariant=Disabled  IntegratorICVariant=Disabled  ExternalResetVariant=Disabled  TRSumVariant=Passthrough  SumFdbkVariant=Disabled  SumVariant=Passthrough_P  TsampFilterVariant=InternalTs  TsampNgainVariant=Passthrough  TsampIntegralVariant=Disabled_SignalSpec  ExternalSaturationOutDataTypeStr=Inherit: Same as second input
  P_yaw : slpidlib/PID Controller  Controller=P  Form=Parallel  TimeDomain=Discrete-time  UseExternalTs=off  SampleTime=-1  IntegratorMethod=Forward Euler  FilterMethod=Forward Euler  ControllerParametersSource=internal  P=1.2  I=0  D=0  UseFilter=on  N=100  TunerSelectOption=Transfer Function Based (PID Tuner App)  InitialConditionSource=internal  InitialConditionForIntegrator=0  InitialConditionForFilter=0  DifferentiatorICPrevScaledInput=0  ExternalReset=none  TrackingMode=off  Kt=1  LimitOutput=off  SatLimitsSource=internal  UpperSaturationLimit=inf  LowerSaturationLimit=-inf  LinearizeAsGain=on  AntiWindupMode=none  Kb=1  POutMin=[]  POutMax=[]  IOutMin=[]  IOutMax=[]  DOutMin=[]  DOutMax=[]  NOutMin=[]  NOutMax=[]  SumOutMin=[]  SumOutMax=[]  SaturationOutMin=[]  SaturationOutMax=[]  PParamMin=[]  PParamMax=[]  IParamMin=[]  IParamMax=[]  DParamMin=[]  DParamMax=[]  NParamMin=[]  NParamMax=[]  KbParamMin=[]  KbParamMax=[]  KtParamMin=[]  KtParamMax=[]  KbOutMin=[]  KbOutMax=[]  KtOutMin=[]  KtOutMax=[]  IntegratorOutMin=[]  IntegratorOutMax=[]  FilterOutMin=[]  FilterOutMax=[]  SumI1OutMin=[]  SumI1OutMax=[]  SumI2OutMin=[]  SumI2OutMax=[]  SumI3OutMin=[]  SumI3OutMax=[]  SumI4OutMin=[]  SumI4OutMax=[]  SumDOutMin=[]  SumDOutMax=[]  DifferentiatorOutMin=[]  DifferentiatorOutMax=[]  FilterDiffOutCoefMin=[]  FilterDiffOutCoefMax=[]  ReciprocalOutMin=[]  ReciprocalOutMax=[]  SumDenOutMin=[]  SumDenOutMax=[]  SumNumOutMin=[]  SumNumOutMax=[]  DivideOutMin=[]  DivideOutMax=[]  UdiffTsProdOutMin=[]  UdiffTsProdOutMax=[]  NTsProdOutMin=[]  NTsProdOutMax=[]  UintegralTsProdOutMin=[]  UintegralTsProdOutMax=[]  UngainTsProdOutMin=[]  UngainTsProdOutMax=[]  IntegratorContinuousStateAttributes=''  IntegratorStateMustResolveToSignalObject=off  IntegratorRTWStateStorageClass=Auto  FilterContinuousStateAttributes=''  FilterStateMustResolveToSignalObject=off  FilterRTWStateStorageClass=Auto  ParallelPVariant=InternalParameters  IdealPVariant=Disabled  IVariant=Disabled  DVariant=Disabled  IntegratorVariant=Disabled  SatVariant=Disabled  AWVariant=Disabled  PCopyVariant=Disabled  TRVariant=Disabled  FdbkBlocksVariant=Forward  IdealPFdbkVariant=Disabled  SatFdbkVariant=Disabled  DerivativeFilterVariant=Disabled  NVariant=Disabled  NCopyVariant=Disabled_SignalSpec  FilterICVariant=Disabled  IntegratorICVariant=Disabled  ExternalResetVariant=Disabled  TRSumVariant=Passthrough  SumFdbkVariant=Disabled  SumVariant=Passthrough_P  TsampFilterVariant=InternalTs  TsampNgainVariant=Passthrough  TsampIntegralVariant=Disabled_SignalSpec  ExternalSaturationOutDataTypeStr=Inherit: Same as second input
  Rotation Angles to Direction Cosine Matrix : sharedtransform/Rotation Angles to Direction Cosine Matrix  rotationOrder=XYZ  aMode=aMode
      settings: SourceProductBaseCode=AE,PW,MT,UV,VE,VP
  Terminator : Terminator
  Transpose : Math  Operator=transpose  SaturateOnIntegerOverflow=on
  offset w_dot by g : Sum
  pitch_setpoint : Constant  Value=0.2*pi/180
  pitch_unwrap : Subsystem
  roll_unwrap : Subsystem
  transform to XYD : Product  Multiplication=Matrix(*)
  v_dot as P setpoint : Selector  InputPortWidth=3  IndexOptions=Index vector (dialog)  Indices=[2]  OutputSizes=1
  yaw_setpoint : Subsystem
  yaw_unwrap : Subsystem
  acc_cmd : Outport
  DEBUG : Outport  Port=2
  wires:
  Mux1/1 -> acc_cmd/1  "acc_cmd"
  P_r/1 -> Mux5/3
  Mux6/1 -> Add1/2  "uvw_dot.state"
  Demux/1 -> Mux/1  "u_dot.desired"
  offset w_dot by g/1 -> Mux6/3
  Add3/1 -> Demux3/1  "pqr.error"
  Demux2/3 -> offset w_dot by g/1
  Add2/1 -> P_w/1  "w.error"
  Demux3/2 -> P_q/1
  P_p/1 -> Mux5/1
  Demux/4 -> yaw_setpoint/1(r_desired)  "r.desired"
  Demux1/3 -> PI_w_dot/1
  Constant1/1 -> offset w_dot by g/2
  Demux/2 -> Mux/2  "v_dot.desired"
  P_w/1 -> Mux/3  "w_dot.desired"
  Mux4/1 -> v_dot as P setpoint/1, Mux1/1  "uvw_dot.cmd"
  Demux3/3 -> P_r/1
  z_vel (NED)/1 -> Add2/2  "w.state"
  Demux3/1 -> P_p/1
  PI_w_dot/1 -> Mux4/3
  P_q/1 -> Mux5/2
  gyro [rad/s] (BF)/1 -> Add3/2  "pqr.state"
  euler [rad] (up pos)/1 -> Add5/2, yaw_setpoint/2(rollpitchyaw.state), Demux5/1  "rollpitchyaw.state"
  PI_u_dot/1 -> Mux4/1
  Demux1/2 -> P_v_dot/1
  Mux/1 -> Add1/1  "uvw_dot.desired"
  RC/1 -> Demux/1
  Mux5/1 -> Mux1/2  "pqr_dot.cmd"
  Add5/1 -> Demux4/1  "rpy.error"
  Add1/1 -> Demux1/1  "uvw_dot.error"
  acc (BF)/1 -> transform to XYD/2  "m/s²"
  Demux/3 -> Add2/1  "w.desired"
  Demux4/2 -> pitch_unwrap/1(theta)
  P_roll/1 -> Mux3/1
  Demux1/1 -> PI_u_dot/1
  Mux3/1 -> Add3/1  "pqr.desired"
  P_pitch/1 -> Mux3/2
  pitch_setpoint/1 -> Mux7/2
  Mux7/1 -> Add5/1
  Demux5/1 -> Mux8/1
  Demux5/2 -> Mux8/2
  Demux5/3 -> Terminator/1
  Constant/1 -> Mux8/3
  Mux8/1 -> Rotation Angles to Direction Cosine Matrix/1
  transform to XYD/1 -> Demux2/1
  Demux2/2 -> Mux6/2
  yaw_setpoint/1(yaw_setpoint) -> Mux7/3
  Demux4/3 -> yaw_unwrap/1(psi)
  P_yaw/1 -> Mux3/3
  yaw_unwrap/1(psi.fix) -> P_yaw/1
  Demux4/1 -> roll_unwrap/1(phi)
  P_v_dot/1 -> Mux4/2
  Demux2/1 -> Mux6/1
  v_dot as P setpoint/1 -> Mux7/1
  Constant2/1 -> DEBUG/1
  Rotation Angles to Direction Cosine Matrix/1 -> Transpose/1
  Transpose/1 -> transform to XYD/1
  pitch_unwrap/1(theta.fix) -> P_pitch/1
  roll_unwrap/1(phi.fix) -> P_roll/1

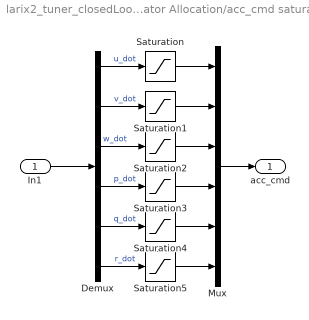
== system larix2_tuner_closedLoop/Actuator Allocation/acc_cmd saturation ==
  In1 : Inport
  Demux : Demux  Outputs=6
  Mux : Mux  Inputs=6
  Saturation : Saturate  UpperLimit=blimp.prp.du_max  LowerLimit=-blimp.prp.du_max
  Saturation1 : Saturate  UpperLimit=blimp.prp.dv_max  LowerLimit=-blimp.prp.dv_max
  Saturation2 : Saturate  UpperLimit=blimp.prp.dw_max  LowerLimit=-blimp.prp.dw_max
  Saturation3 : Saturate  UpperLimit=blimp.prp.dp_max  LowerLimit=-blimp.prp.dp_max
  Saturation4 : Saturate  UpperLimit=blimp.prp.dq_max  LowerLimit=-blimp.prp.dq_max
  Saturation5 : Saturate  UpperLimit=blimp.prp.dr_max  LowerLimit=-blimp.prp.dr_max
  acc_cmd : Outport
  wires:
  In1/1 -> Demux/1
  Mux/1 -> acc_cmd/1
  Demux/1 -> Saturation/1  "u_dot"
  Saturation/1 -> Mux/1
  Demux/2 -> Saturation1/1  "v_dot"
  Saturation1/1 -> Mux/2
  Demux/3 -> Saturation2/1  "w_dot"
  Saturation2/1 -> Mux/3
  Demux/4 -> Saturation3/1  "p_dot"
  Saturation3/1 -> Mux/4
  Demux/5 -> Saturation4/1  "q_dot"
  Saturation4/1 -> Mux/5
  Demux/6 -> Saturation5/1  "r_dot"
  Saturation5/1 -> Mux/6

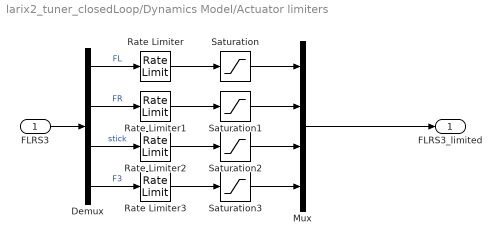
== system larix2_tuner_closedLoop/Dynamics Model/Actuator limiters ==
  FLRS3 : Inport
  Demux : Demux
  Mux : Mux
  Rate Limiter : RateLimiter  RisingSlewLimit=blimp.prp.dFLR_max  FallingSlewLimit=-blimp.prp.dFLR_max  SampleTimeMode=inherited
  Rate Limiter1 : RateLimiter  RisingSlewLimit=blimp.prp.dFLR_max  FallingSlewLimit=-blimp.prp.dFLR_max  SampleTimeMode=inherited
  Rate Limiter2 : RateLimiter  RisingSlewLimit=blimp.prp.dstick_max  FallingSlewLimit=-blimp.prp.dstick_max  SampleTimeMode=inherited
  Rate Limiter3 : RateLimiter  RisingSlewLimit=blimp.prp.dF3_max  FallingSlewLimit=-blimp.prp.dF3_max  SampleTimeMode=inherited
  Saturation : Saturate  UpperLimit=blimp.prp.FL_max  LowerLimit=blimp.prp.FL_min
  Saturation1 : Saturate  UpperLimit=blimp.prp.FR_max  LowerLimit=blimp.prp.FR_min
  Saturation2 : Saturate  UpperLimit=blimp.prp.stick_max  LowerLimit=blimp.prp.stick_min
  Saturation3 : Saturate  UpperLimit=blimp.prp.FB_max  LowerLimit=blimp.prp.FB_min
  FLRS3_limited : Outport
  wires:
  FLRS3/1 -> Demux/1
  Demux/1 -> Rate Limiter/1  "FL"
  Rate Limiter/1 -> Saturation/1
  Demux/2 -> Rate Limiter1/1  "FR"
  Rate Limiter1/1 -> Saturation1/1
  Demux/3 -> Rate Limiter2/1  "stick"
  Rate Limiter2/1 -> Saturation2/1
  Demux/4 -> Rate Limiter3/1  "F3"
  Rate Limiter3/1 -> Saturation3/1
  Mux/1 -> FLRS3_limited/1
  Saturation/1 -> Mux/1
  Saturation1/1 -> Mux/2
  Saturation2/1 -> Mux/3
  Saturation3/1 -> Mux/4

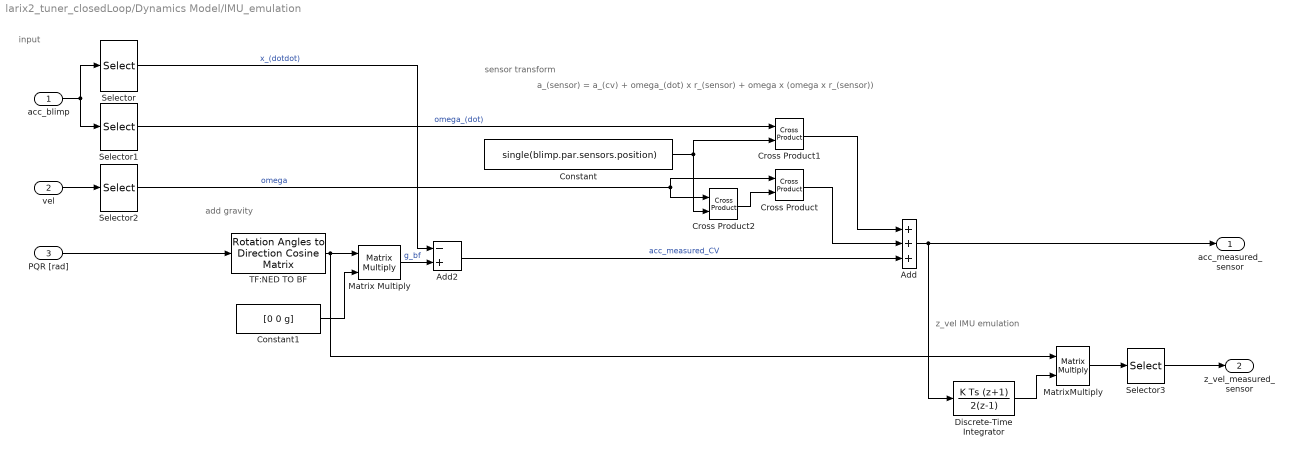
== system larix2_tuner_closedLoop/Dynamics Model/IMU_emulation ==
  note: z_vel IMU emulation
  note: a_(sensor) = a_(cv) + omega_(dot) x r_(sensor) + omega x (omega x r_(sensor))
  note: input
  note: add gravity
  note: sensor transform
  acc_blimp : Inport
  vel : Inport  Port=2
  PQR [rad] : Inport  Port=3
  Add : Sum  Inputs=+++
  Add2 : Sum  Inputs=-+
  Constant : Constant  Value=single(blimp.par.sensors.position)
  Constant1 : Constant  Value=[0 0 g]
  Cross Product : vrlib/Utilities/Cross Product
  Cross Product1 : vrlib/Utilities/Cross Product
  Cross Product2 : vrlib/Utilities/Cross Product
  Discrete-Time Integrator : DiscreteIntegrator  IntegratorMethod=Integration: Trapezoidal  gainval=1  SampleTime=-1  ICPrevOutput=DiscIntNeverNeededParam  ICPrevScaledInput=DiscIntNeverNeededParam
  Matrix Multiply : Product  Multiplication=Matrix(*)
  MatrixMultiply : Product  Multiplication=Matrix(*)
  Selector : Selector  InputPortWidth=6  IndexOptions=Index vector (dialog)  Indices=[1 2 3]  OutputSizes=1
  Selector1 : Selector  InputPortWidth=6  IndexOptions=Index vector (dialog)  Indices=[4 5 6]  OutputSizes=1
  Selector2 : Selector  InputPortWidth=6  IndexOptions=Index vector (dialog)  Indices=[4 5 6]  OutputSizes=1
  Selector3 : Selector  InputPortWidth=3  IndexOptions=Index vector (dialog)  Indices=[3]  OutputSizes=1
  TF:NED TO BF : sharedtransform/Rotation Angles to Direction Cosine Matrix  rotationOrder=XYZ  aMode=aMode
      settings: SourceProductBaseCode=AE,PW,MT,UV,VE,VP
  acc_measured_sensor : Outport
  z_vel_measured_sensor : Outport  Port=2
  wires:
  Add2/1 -> Add/3  "acc_measured_CV"
  Cross Product/1 -> Add/2
  Cross Product2/1 -> Cross Product/2
  Cross Product1/1 -> Add/1
  Selector/1 -> Add2/1  "x_(dotdot)"
  Constant/1 -> Cross Product1/2, Cross Product2/2
  acc_blimp/1 -> Selector1/1, Selector/1
  Constant1/1 -> Matrix Multiply/2
  Matrix Multiply/1 -> Add2/2  "g_bf"
  TF:NED TO BF/1 -> MatrixMultiply/1, Matrix Multiply/1
  PQR [rad]/1 -> TF:NED TO BF/1
  Selector1/1 -> Cross Product1/1  "omega_(dot)"
  vel/1 -> Selector2/1
  Selector2/1 -> Cross Product/1, Cross Product2/1  "omega"
  Add/1 -> Discrete-Time Integrator/1, acc_measured_sensor/1
  Discrete-Time Integrator/1 -> MatrixMultiply/2
  MatrixMultiply/1 -> Selector3/1
  Selector3/1 -> z_vel_measured_sensor/1

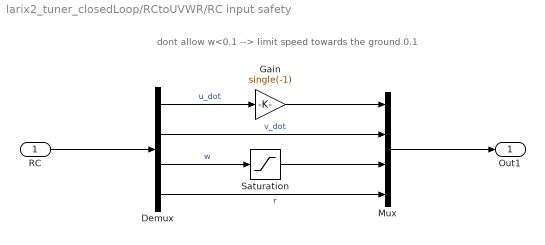
== system larix2_tuner_closedLoop/RCtoUVWR/RC input safety ==
  note: dont allow w<0.1 --> limit speed towards the ground
      |
      |  0.1
  RC : Inport
  Demux : Demux
  Gain : Gain  Gain=single(-1)
  Mux : Mux
  Saturation : Saturate  UpperLimit=1  LowerLimit=-0.2
  Out1 : Outport
  wires:
  RC/1 -> Demux/1
  Mux/1 -> Out1/1
  Demux/1 -> Gain/1  "u_dot"
  Demux/2 -> Mux/2  "v_dot"
  Demux/4 -> Mux/4  "r"
  Demux/3 -> Saturation/1  "w"
  Saturation/1 -> Mux/3
  Gain/1 -> Mux/1

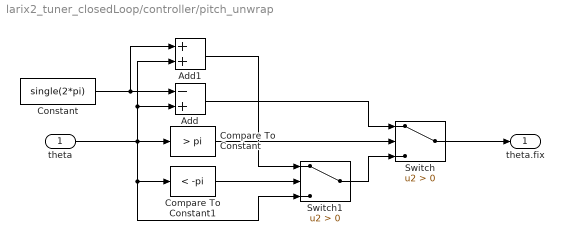
== system larix2_tuner_closedLoop/controller/pitch_unwrap ==
  theta : Inport
  Add : Sum  Inputs=-+
  Add1 : Sum
  Compare To Constant : simulink/Logic and Bit Operations/Compare To Constant  relop=>  const=pi  OutDataTypeStr=boolean
  Compare To Constant1 : simulink/Logic and Bit Operations/Compare To Constant  relop=<  const=-pi  OutDataTypeStr=boolean
  Constant : Constant  Value=single(2*pi)
  Switch : Switch  Criteria=u2 > Threshold
  Switch1 : Switch  Criteria=u2 > Threshold
  theta.fix : Outport
  wires:
  theta/1 -> Switch1/3, Compare To Constant1/1, Compare To Constant/1, Add1/2, Add/2
  Compare To Constant/1 -> Switch/2
  Constant/1 -> Add/1, Add1/1
  Add/1 -> Switch/1
  Compare To Constant1/1 -> Switch1/2
  Switch/1 -> theta.fix/1
  Switch1/1 -> Switch/3
  Add1/1 -> Switch1/1

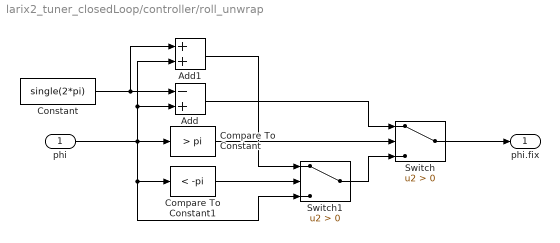
== system larix2_tuner_closedLoop/controller/roll_unwrap ==
  phi : Inport
  Add : Sum  Inputs=-+
  Add1 : Sum
  Compare To Constant : simulink/Logic and Bit Operations/Compare To Constant  relop=>  const=pi  OutDataTypeStr=boolean
  Compare To Constant1 : simulink/Logic and Bit Operations/Compare To Constant  relop=<  const=-pi  OutDataTypeStr=boolean
  Constant : Constant  Value=single(2*pi)
  Switch : Switch  Criteria=u2 > Threshold
  Switch1 : Switch  Criteria=u2 > Threshold
  phi.fix : Outport
  wires:
  phi/1 -> Switch1/3, Compare To Constant1/1, Compare To Constant/1, Add1/2, Add/2
  Compare To Constant/1 -> Switch/2
  Constant/1 -> Add/1, Add1/1
  Add/1 -> Switch/1
  Compare To Constant1/1 -> Switch1/2
  Switch/1 -> phi.fix/1
  Switch1/1 -> Switch/3
  Add1/1 -> Switch1/1

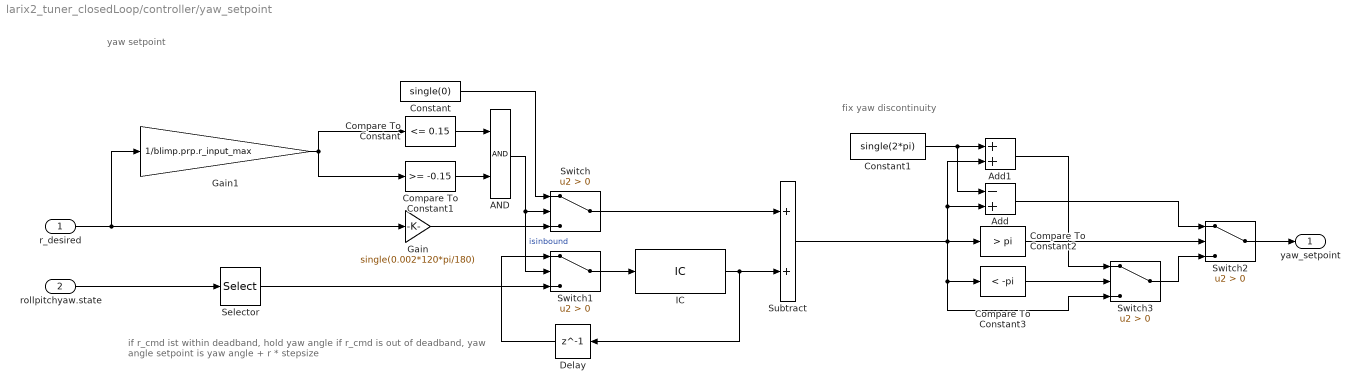
== system larix2_tuner_closedLoop/controller/yaw_setpoint ==
  note: fix yaw discontinuity
  note: yaw setpoint
  note: if r_cmd ist within deadband, hold yaw angle
      | if r_cmd is out of deadband, yaw angle setpoint is yaw angle + r * stepsize
  r_desired : Inport
  rollpitchyaw.state : Inport  Port=2
  AND : Logic  AllPortsSameDT=off  OutDataTypeStr=boolean
  Add : Sum  Inputs=-+
  Add1 : Sum
  Compare To Constant : simulink/Logic and Bit Operations/Compare To Constant  relop=<=  const=0.15  OutDataTypeStr=boolean
  Compare To Constant1 : simulink/Logic and Bit Operations/Compare To Constant  relop=>=  const=-0.15  OutDataTypeStr=boolean
  Compare To Constant2 : simulink/Logic and Bit Operations/Compare To Constant  relop=>  const=pi  OutDataTypeStr=boolean
  Compare To Constant3 : simulink/Logic and Bit Operations/Compare To Constant  relop=<  const=-pi  OutDataTypeStr=boolean
  Constant : Constant  Value=single(0)
  Constant1 : Constant  Value=single(2*pi)
  Delay : Delay  DelayLength=1
  Gain : Gain  Gain=single(0.002*120*pi/180)
  Gain1 : Gain  Gain=1/blimp.prp.r_input_max
  IC : InitialCondition  Value=single(eul_0(3))
  Selector : Selector  InputPortWidth=3  IndexOptions=Index vector (dialog)  Indices=[3]  OutputSizes=1
  Subtract : Sum
  Switch{,1..3} (4 alike) : Switch  Criteria=u2 > Threshold
  yaw_setpoint : Outport
  wires:
  r_desired/1 -> Gain/1, Gain1/1
  Compare To Constant/1 -> AND/1
  Compare To Constant1/1 -> AND/2
  AND/1 -> Switch/2, Switch1/2  "isinbound"
  Constant/1 -> Switch/1
  Switch/1 -> Subtract/1
  rollpitchyaw.state/1 -> Selector/1
  Selector/1 -> Switch1/3
  Switch1/1 -> IC/1
  Gain/1 -> Switch/3
  Gain1/1 -> Compare To Constant1/1, Compare To Constant/1
  Delay/1 -> Switch1/1
  IC/1 -> Delay/1, Subtract/2
  Subtract/1 -> Switch3/3, Compare To Constant3/1, Compare To Constant2/1, Add1/2, Add/2
  Add1/1 -> Switch3/1
  Compare To Constant3/1 -> Switch3/2
  Constant1/1 -> Add1/1, Add/1
  Switch2/1 -> yaw_setpoint/1
  Add/1 -> Switch2/1
  Compare To Constant2/1 -> Switch2/2
  Switch3/1 -> Switch2/3

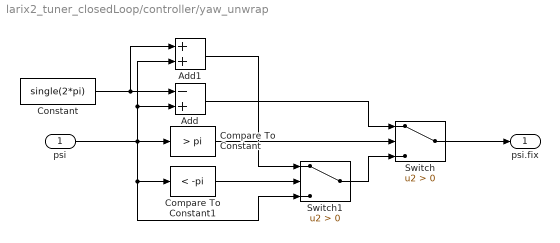
== system larix2_tuner_closedLoop/controller/yaw_unwrap ==
  psi : Inport
  Add : Sum  Inputs=-+
  Add1 : Sum
  Compare To Constant : simulink/Logic and Bit Operations/Compare To Constant  relop=>  const=pi  OutDataTypeStr=boolean
  Compare To Constant1 : simulink/Logic and Bit Operations/Compare To Constant  relop=<  const=-pi  OutDataTypeStr=boolean
  Constant : Constant  Value=single(2*pi)
  Switch : Switch  Criteria=u2 > Threshold
  Switch1 : Switch  Criteria=u2 > Threshold
  psi.fix : Outport
  wires:
  psi/1 -> Switch1/3, Compare To Constant1/1, Compare To Constant/1, Add1/2, Add/2
  Compare To Constant/1 -> Switch/2
  Constant/1 -> Add/1, Add1/1
  Add/1 -> Switch/1
  Compare To Constant1/1 -> Switch1/2
  Switch/1 -> psi.fix/1
  Switch1/1 -> Switch/3
  Add1/1 -> Switch1/1
